simulink model "progetto_simulink_new"  (R2019b)
settings: Solver=VariableStepAuto  StartTime=0.0  StopTime=100  RelTol=1e-3
values from neighbouring files (symbols this model uses):
  DenL = DenL{1,1}    [progetto_3A.m]    (also in progetto_3A_new.m; progetto_3A_new_utf8.m; progetto_3A_piano_B.m; progetto_3A_piano_B_utf8.m)
  DenR = DenR{1,1}    [progetto_3A.m]    (also in progetto_3A_new.m; progetto_3A_new_utf8.m; progetto_3A_piano_B.m; progetto_3A_piano_B_utf8.m)
  NumL = NumL{1,1}    [progetto_3A.m]    (also in progetto_3A_new.m; progetto_3A_new_utf8.m; progetto_3A_piano_B.m; progetto_3A_piano_B_utf8.m)
  NumR = NumR{1,1}    [progetto_3A.m]    (also in progetto_3A_new.m; progetto_3A_new_utf8.m; progetto_3A_piano_B.m; progetto_3A_piano_B_utf8.m)
undefined symbols (not defined in the file or in its folder): DenG, NumG, tab
settings Model: Creator=Luca  LastModifiedBy=luca

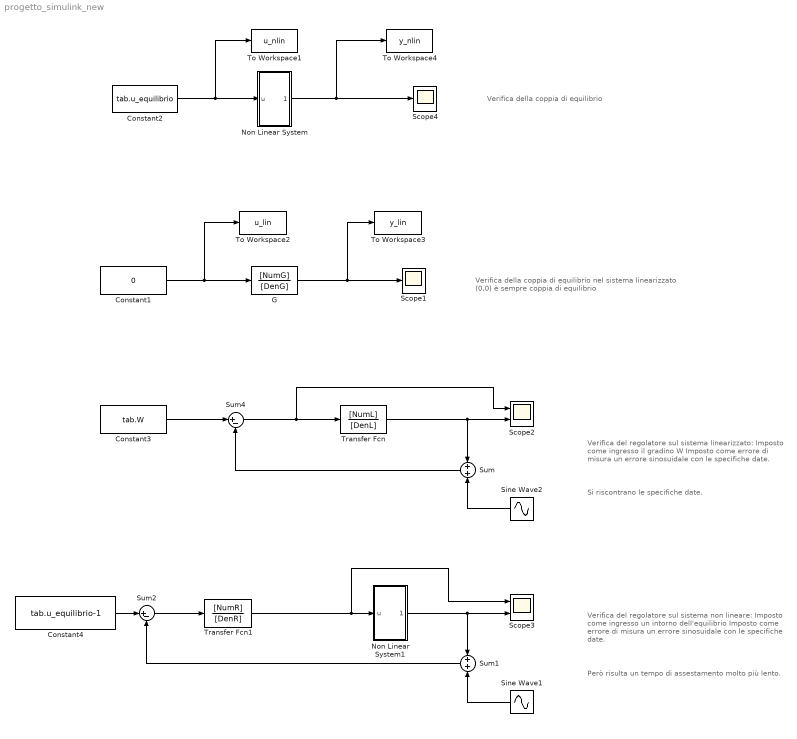
== system progetto_simulink_new ==
  note: Però risulta un tempo di assestamento molto più lento.
  note: Si riscontrano le specifiche date.
  note: Verifica del regolatore sul sistema linearizzato:
      | Imposto come ingresso il gradino W
      | Imposto come errore di misura un errore sinosuidale
      | con le specifiche date.
  note: Verifica della coppia di equilibrio
  note: Verifica della coppia di equilibrio nel sistema linearizzato
      | (0,0) è sempre coppia di equilibrio
  note: Verifica del regolatore sul sistema non lineare:
      | Imposto come ingresso un intorno dell'equilibrio
      | Imposto come errore di misura un errore sinosuidale
      | con le specifiche date.
  Constant1 : Constant  Value=0
  Constant2 : Constant  Value=tab.u_equilibrio
  Constant3 : Constant  Value=tab.W
  Constant4 : Constant  Value=tab.u_equilibrio-1
  G : TransferFcn  Numerator=[NumG]  Denominator=[DenG]
  Non Linear System : Subsystem
  Non Linear System1 : Subsystem
  Scope1 : Scope
  Scope2 : Scope  NumInputPorts=2
  Scope3 : Scope  NumInputPorts=2
  Scope4 : Scope
  Sine Wave1 : Sin  Amplitude=tab.A_n  Frequency=tab.omega_n  SampleTime=0
  Sine Wave2 : Sin  Amplitude=tab.A_n  Frequency=tab.omega_n  SampleTime=0
  Sum : Sum  Inputs=2
  Sum1 : Sum  Inputs=2
  Sum2 : Sum  Inputs=|+-
  Sum4 : Sum  Inputs=|+-
  To Workspace1 : ToWorkspace  VariableName=u_nlin  SaveFormat=Timeseries  SampleTime=-1
  To Workspace2 : ToWorkspace  VariableName=u_lin  SaveFormat=Timeseries  SampleTime=-1
  To Workspace3 : ToWorkspace  VariableName=y_lin  SaveFormat=Timeseries  SampleTime=-1
  To Workspace4 : ToWorkspace  VariableName=y_nlin  SaveFormat=Timeseries  SampleTime=-1
  Transfer Fcn : TransferFcn  Numerator=[NumL]  Denominator=[DenL]
  Transfer Fcn1 : TransferFcn  Numerator=[NumR]  Denominator=[DenR]
  wires:
  Constant2/1 -> Non Linear System/1(u), To Workspace1/1
  G/1 -> To Workspace3/1, Scope1/1
  Constant1/1 -> G/1, To Workspace2/1
  Non Linear System/1(Out1) -> To Workspace4/1, Scope4/1
  Sum4/1 -> Scope2/1, Transfer Fcn/1
  Transfer Fcn/1 -> Sum/1, Scope2/2
  Sum/1 -> Sum4/2
  Constant3/1 -> Sum4/1
  Sine Wave2/1 -> Sum/2
  Constant4/1 -> Sum2/1
  Sum1/1 -> Sum2/2
  Sine Wave1/1 -> Sum1/2
  Non Linear System1/1(Out1) -> Sum1/1, Scope3/2
  Sum2/1 -> Transfer Fcn1/1
  Transfer Fcn1/1 -> Scope3/1, Non Linear System1/1(u)

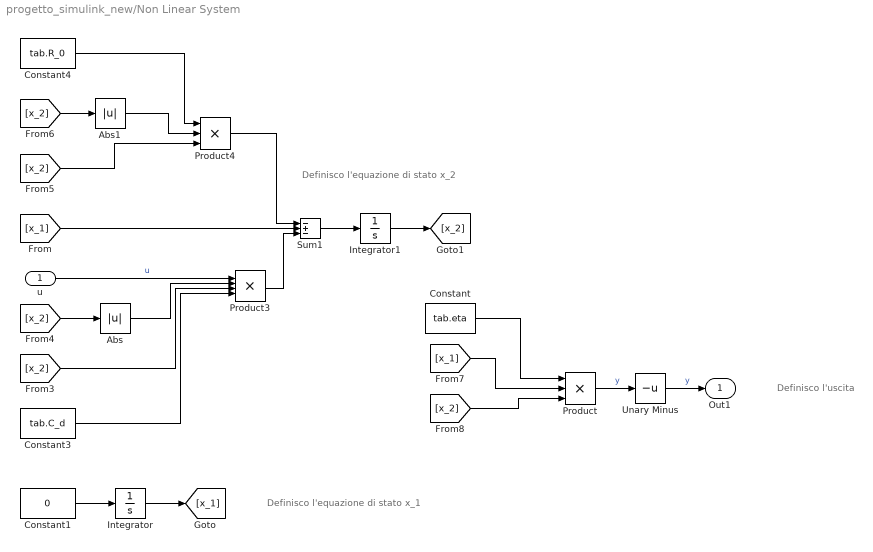
== system progetto_simulink_new/Non Linear System ==
  note: Definisco l'uscita
  note: Definisco l'equazione di stato x_1
  note: Definisco l'equazione di stato x_2
  u : Inport
  Abs : Abs
  Abs1 : Abs
  Constant : Constant  Value=tab.eta
  Constant1 : Constant  Value=0
  Constant3 : Constant  Value=tab.C_d
  Constant4 : Constant  Value=tab.R_0
  Integrator : Integrator  InitialCondition=tab.x_equilibrio_1
  Integrator1 : Integrator  InitialCondition=tab.x_equilibrio_2
  Product : Product  Inputs=3
  Product3 : Product  Inputs=4
  Product4 : Product  Inputs=3
  Sum1 : Sum  Inputs=-+-
  Unary Minus : UnaryMinus
  Out1 : Outport
  wires:
  Integrator/1 -> [x_1]
  Integrator1/1 -> [x_2]
  Product3/1 -> Sum1/3
  Constant1/1 -> Integrator/1
  [x_2] -> Product/3
  Constant3/1 -> Product3/4
  [x_1] -> Product/2
  Sum1/1 -> Integrator1/1
  Abs1/1 -> Product4/2
  [x_1] -> Sum1/2
  [x_2] -> Abs/1
  Product/1 -> Unary Minus/1  "y"
  Constant4/1 -> Product4/1
  Abs/1 -> Product3/2
  [x_2] -> Product3/3
  u/1 -> Product3/1  "u"
  [x_2] -> Abs1/1
  [x_2] -> Product4/3
  Product4/1 -> Sum1/1
  Constant/1 -> Product/1
  Unary Minus/1 -> Out1/1  "y"

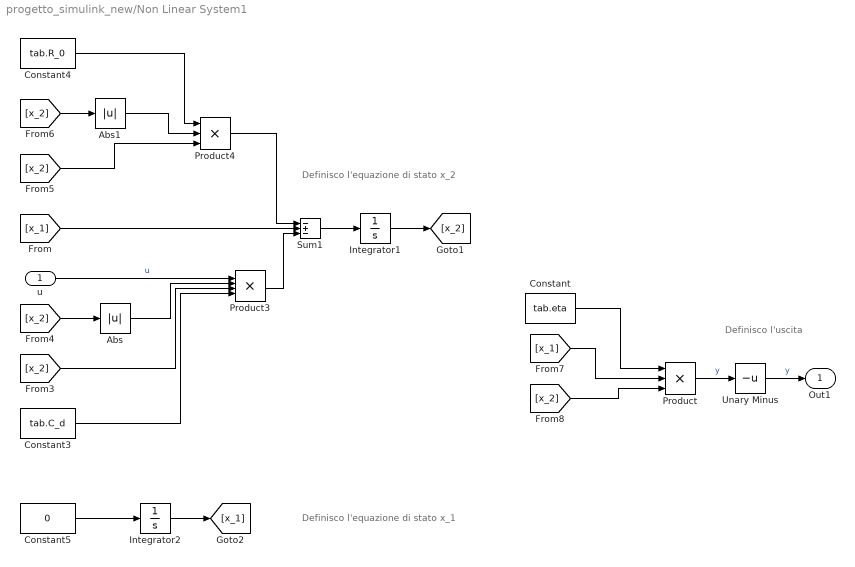
== system progetto_simulink_new/Non Linear System1 ==
  note: Definisco l'uscita
  note: Definisco l'equazione di stato x_1
  note: Definisco l'equazione di stato x_2
  u : Inport
  Abs : Abs
  Abs1 : Abs
  Constant : Constant  Value=tab.eta
  Constant3 : Constant  Value=tab.C_d
  Constant4 : Constant  Value=tab.R_0
  Constant5 : Constant  Value=0
  Integrator1 : Integrator  InitialCondition=tab.x_equilibrio_2
  Integrator2 : Integrator  InitialCondition=tab.x_equilibrio_1
  Product : Product  Inputs=3
  Product3 : Product  Inputs=4
  Product4 : Product  Inputs=3
  Sum1 : Sum  Inputs=-+-
  Unary Minus : UnaryMinus
  Out1 : Outport
  wires:
  Integrator1/1 -> [x_2]
  Product3/1 -> Sum1/3
  [x_2] -> Product/3
  Constant3/1 -> Product3/4
  [x_1] -> Product/2
  Sum1/1 -> Integrator1/1
  Abs1/1 -> Product4/2
  Integrator2/1 -> [x_1]
  [x_1] -> Sum1/2
  [x_2] -> Abs/1
  Product/1 -> Unary Minus/1  "y"
  Constant4/1 -> Product4/1
  Abs/1 -> Product3/2
  [x_2] -> Product3/3
  u/1 -> Product3/1  "u"
  [x_2] -> Abs1/1
  [x_2] -> Product4/3
  Product4/1 -> Sum1/1
  Constant/1 -> Product/1
  Unary Minus/1 -> Out1/1  "y"
  Constant5/1 -> Integrator2/1
